simulink model "TimeSyncTest"  (R2016b)
settings: Solver=ode4  StartTime=0.0  StopTime=inf  FixedStep=0.001  RelTol=1e-3  EnableMultiTasking=on
libraries: robotlib x2, sldrtlib x1
Description:
  | Real-Time Van der Pol Simulation
  | 
  | The example model "sldrtex_vdp" shows a real-time version of the Simulink(R) Van der Pol
  | simulation model. This model does not need any external signals, so it does
  | not need any data acquisition hardware or driver. This makes the model ideal
  | for the first experiments with Simulink Desktop Real-Time(TM), without need to
  | worry about proper I/O hardware configuration.
  | 
  | How to run this model in Normal Mode:
  | 
  | 1) Double-click the orange button to switch to Normal Mode if needed.
  | 2) Start the real-time execution using Simulation->Run.
  | 3) Observe any missed ticks on the Missed Ticks scope.
  | 
  | How to run this model in External Mode:
  | 
  | 1) Double-click the orange button to switch to External Mode if needed.
  | 2) Start the real-time execution using Simulation->Run. The model will automatically
  |    build, connect to Simulink in External Mode and start.
  | 3) Missed ticks will be always zero.
settings Model: ExtModeTrigDuration=101  Creator=The MathWorks, Inc.  LastModifiedBy=shangguanlantian
settings DataIOCC: LimitDataPoints=on  SaveFormat=Array  SignalLoggingName=logsOut
settings OptimizationCC: ExpressionDepthLimit=2147483647  InitFltsAndDblsToZero=on  EfficientMapNaN2IntZero=off  LifeSpan=inf
settings DebuggingCC: UnderspecifiedInitializationDetection=Classic  MergeDetectMultiDrivingBlocksExec=none  SignalResolutionControl=TryResolveAllWithWarning  FcnCallInpInsideContextMsg=warning  AllowSymbolicDim=off  StateNameClashWarn=warning  SFUnexpectedBacktrackingDiag=warning  SFNoUnconditionalDefaultTransitionDiag=warning  SFExecutionAtInitializationDiag=none
settings HardwareCC: TargetBitPerLong=64  TargetBitPerPointer=64  TargetBitPerSizeT=64  TargetBitPerPtrDiffT=64  TargetIntDivRoundTo=Zero  TargetEndianess=LittleEndian  TargetWordSize=64  TargetHWDeviceType=Intel->x86-64
settings ModelReferenceCC: PropagateSignalLabelsOutOfModel=off
settings RTWCC: SystemTargetFile=sldrt.tlc  TemplateMakefile=sldrt.tmf  Description=Simulink Desktop Real-Time  RTWCompilerOptimization=on
settings CodeAppCC: MaxIdLength=95
settings SimulinkDesktopRealTimeCC: TargetPreCompLibLocation=C:\Program Files\MATLAB\R2016B\toolbox\sldrt\lib\win64  TargetLangStandard=C89/C90 (ANSI)  GeneratePreprocessorConditionals=Disable all  SupportVariableSizeSignals=off
settings ConfigComp: CovMetricSettings=dw  CovHtmlReporting=on  CovSaveCumulativeToWorkspaceVar=on  CovSaveSingleToWorkspaceVar=on  CovShowResultsExplorer=off  CovExternalEMLEnable=off  CovSFcnEnable=off

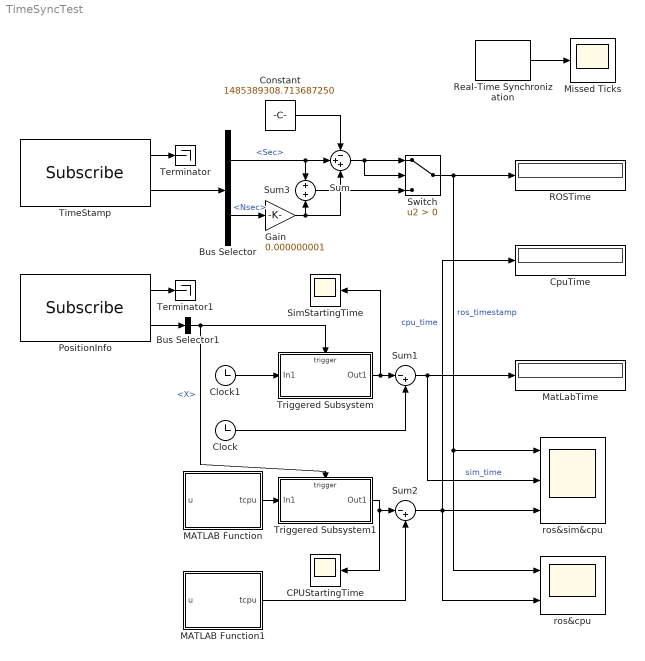
== system TimeSyncTest ==
  Bus Selector : BusSelector  OutputSignals=Header.Stamp.Sec,Header.Stamp.Nsec
  Bus Selector1 : BusSelector  OutputSignals=Pose.Position.X
  CPUStartingTime : Scope
  Clock : Clock
  Clock1 : Clock
  Constant : Constant  Value=1485389308.713687250
  CpuTime : Display
  Gain : Gain  Gain=0.000000001
  MATLAB Function : MATLAB Function  TreatAsAtomicUnit=on
  MATLAB Function1 : MATLAB Function  TreatAsAtomicUnit=on
  MatLabTime : Display
  Missed Ticks : Scope
  PositionInfo : robotlib/Subscribe  SourceLibraryInfo=This block requires Robotics System Toolbox  topicSource=Select from ROS network  topic=/slam_out_pose  messageType=geometry_msgs/PoseStamped  sampleTime=-1  messageQueueLength=1
  ROSTime : Display
  Real-Time Synchronization : sldrtlib/Real-Time Synchronization  SampleTime=0.1  MaxMissedTicks=100000  ShowMissedTicks=on  YieldWhenWaiting=off
  SimStartingTime : Scope
  Sum : Sum  Inputs=-++
  Sum1 : Sum  Inputs=|-+
  Sum2 : Sum  Inputs=|-+
  Sum3 : Sum
  Switch : Switch  Criteria=u2 > Threshold
  Terminator : Terminator
  Terminator1 : Terminator
  TimeStamp : robotlib/Subscribe  SourceLibraryInfo=This block requires Robotics System Toolbox  topicSource=Select from ROS network  topic=/slam_out_pose  messageType=geometry_msgs/PoseStamped  sampleTime=-1  messageQueueLength=1
  Triggered Subsystem : Subsystem  TreatAsAtomicUnit=on
  Triggered Subsystem1 : Subsystem  TreatAsAtomicUnit=on
  ros&cpu : Scope  NumInputPorts=2
  ros&sim&cpu : Scope  NumInputPorts=3
  wires:
  Real-Time Synchronization/1 -> Missed Ticks/1
  TimeStamp/1 -> Terminator/1
  TimeStamp/2 -> Bus Selector/1
  Bus Selector/1 -> Sum3/1, Sum/2  "<Sec>"
  Constant/1 -> Sum/1
  Sum/1 -> Switch/1, Switch/2
  Bus Selector/2 -> Gain/1  "<Nsec>"
  Gain/1 -> Sum3/2, Sum/3
  PositionInfo/1 -> Terminator1/1
  PositionInfo/2 -> Bus Selector1/1
  Bus Selector1/1 -> Triggered Subsystem1/Trigger, Triggered Subsystem/Trigger  "<X>"
  Clock/1 -> Sum1/2
  Sum1/1 -> MatLabTime/1, ros&sim&cpu/2  "sim_time"
  Clock1/1 -> Triggered Subsystem/1(In1)
  Triggered Subsystem/1(Out1) -> SimStartingTime/1, Sum1/1
  Sum3/1 -> Switch/3
  Switch/1 -> ROSTime/1, ros&sim&cpu/1, ros&cpu/1  "ros_timestamp"
  Sum2/1 -> ros&sim&cpu/3, ros&cpu/2, CpuTime/1  "cpu_time"
  MATLAB Function/1(tcpu) -> Triggered Subsystem1/1(In1)
  Triggered Subsystem1/1(Out1) -> Sum2/1, CPUStartingTime/1
  MATLAB Function1/1(tcpu) -> Sum2/2

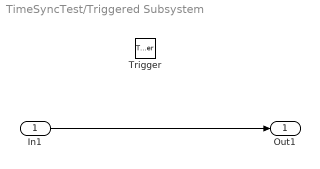
== system TimeSyncTest/Triggered Subsystem ==
  In1 : Inport
  Trigger : TriggerPort  VariantControl=Variant
  Out1 : Outport
  wires:
  In1/1 -> Out1/1

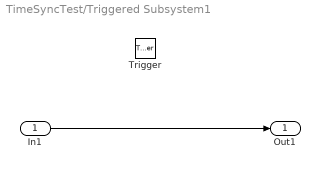
== system TimeSyncTest/Triggered Subsystem1 ==
  In1 : Inport
  Trigger : TriggerPort  VariantControl=Variant
  Out1 : Outport
  wires:
  In1/1 -> Out1/1

== matlab function TimeSyncTest/MATLAB Function ==
  data: u input; tcpu output
function tcpu = fcn(u)
coder.extrinsic('cputime')
persistent t_0
if isempty(t_0)
    t_0 = 0;
    t_0 = cputime;
end
t = 0;
t = cputime;
tcpu = t - t_0;
end

== matlab function TimeSyncTest/MATLAB Function1 ==
  data: u input; tcpu output
function tcpu = fcn(u)
coder.extrinsic('cputime')
persistent t_0
    if isempty(t_0)
    t_0 = 0;
    t_0 = cputime;
    end
t = 0;
t = cputime;
tcpu = t - t_0;
end
